simulink model "PROVA_FINALE_LOAD_ARDUINO_15_10_RIF_COSTANTI"  (R2020b)
settings: Solver=FixedStepDiscrete  StartTime=0.0  StopTime=Inf  FixedStep=0.02  RelTol=1e-3  EnableMultiTasking=on
undefined symbols (not defined in the file or in its folder): attuatore_Amax, attuatore_Amin, attuatore_Emax, attuatore_Emin, attuatore_Rmax, attuatore_Rmin, attuatore_Tmax, attuatore_Tmin, DiscIntNeverNeededParam, interventoA_05, interventoA_1, interventoE_05, interventoE_1, interventoT, inv_A, inv_comp_h, inv_E, inv_R, inv_T, K_AW_B_AP_quota, K_AW_B_becc, K_AW_B_imb, K_AW_B_roll, K_imb_inv, Kd_h_app, Kd_h_flare, Ki_AP_quota_select, Ki_AP_rotta, Ki_AP_vel, Ki_becch, Ki_h_app, Ki_h_cruise, Ki_h_flare, Ki_roll, Kp_AP_quota_hold_h, Kp_AP_quota_hold_l, Kp_AP_quota_select, Kp_AP_rotta, Kp_AP_vel, Kp_becch, Kp_comp_h, Kp_h_app_max, Kp_h_app_min, Kp_h_cruise, Kp_h_flare, Kp_imb, Kp_p, Kp_q, Kp_roll, Kp_Rotta_ATO, Newton, phi_max, phi_min, Raphson, safe_phi, safe_V, t_AP, theta_max, theta_min, time_alarm_SAFE ... (+5)
libraries: simulink_extras x34, arduinolib x24, pid_lib x8, simulink x3, dspsigops x3, svdutilitieslib x3, aerolibtransform2sys x2, aerolibtransform2 x2
(part 2 of 7)

== system PROVA_FINALE_LOAD_ARDUINO_15_10_RIF_COSTANTI/AIR TX/IMU & Attidude ==
  note: NB.: se non si posside un dato inserire una costante con valore 0. I dati vanno messi tutti anche se zeri nell'ordine elencato
  note: Vanno inseriti i collegamenti con i dati provenienti dal sensore inerziale (MTi)
      | in uscita bisogna dare un vettore di 12 componenti contente in ordine:
      | - 3 accelerazioni (x,y,z)
      | - 3 giroscopiche (p,q,r)
      | - 3 comp. campo magnetico
      | -3 angoli di eulero
  AHRS1 : Inport
  Bus Selector : BusSelector  OutputSignals=acc,p,q,r,phi,theta,psi
  Constant : Constant  Value=0  OutDataTypeStr=double  SampleTime=t_AP
  Constant1 : Constant  Value=0  OutDataTypeStr=double  SampleTime=t_AP
  Constant2 : Constant  Value=0  OutDataTypeStr=double  SampleTime=t_AP
  Data Type Conversion : DataTypeConversion  OutDataTypeStr=int16  RndMeth=Simplest
  Data Type Conversion1 : DataTypeConversion  OutDataTypeStr=single
  Gain : Gain  Gain=10^3
  Mux{1,3..5} (4 alike) : Mux  Inputs=3
  Mux2 : Mux  Inputs=2
  IMU : Outport  VectorParamsAs1DForOutWhenUnconnected=off
  ATT : Outport  Port=2  VectorParamsAs1DForOutWhenUnconnected=off
  wires:
  Constant/1 -> Mux5/1
  Mux4/1 -> Mux2/1
  Bus Selector/7 -> Mux4/3  "<psi>"
  Bus Selector/6 -> Mux4/2  "<theta>"
  Bus Selector/5 -> Mux4/1  "<phi>"
  Mux3/1 -> Mux2/2, Mux1/2
  Bus Selector/4 -> Mux3/3  "<r>"
  Bus Selector/3 -> Mux3/2  "<q>"
  Bus Selector/2 -> Mux3/1  "<p>"
  Bus Selector/1 -> Mux1/1  "<acc>"
  AHRS1/1 -> Bus Selector/1
  Mux2/1 -> Data Type Conversion1/1
  Gain/1 -> Data Type Conversion/1
  Data Type Conversion1/1 -> ATT/1
  Data Type Conversion/1 -> IMU/1
  Mux1/1 -> Gain/1
  Constant1/1 -> Mux5/2
  Mux5/1 -> Mux1/3
  Constant2/1 -> Mux5/3

== system PROVA_FINALE_LOAD_ARDUINO_15_10_RIF_COSTANTI/AIR TX/If_subsystem ==
  note: Blocco per la temporizzazione dell'invio dei messaggi
  Data Type Conversion3 : DataTypeConversion  OutDataTypeStr=uint32  RndMeth=Simplest
  Gain : Gain  Gain=100
  Subsystem : Subsystem
  iflogic_function : MATLAB Function  TreatAsAtomicUnit=on
  iflogic : Outport  VectorParamsAs1DForOutWhenUnconnected=off
  time : Outport  Port=2  VectorParamsAs1DForOutWhenUnconnected=off
  wires:
  Subsystem/3(time) -> Gain/1
  Subsystem/2(H_10) -> iflogic_function/2(H10)
  Subsystem/1(H_50) -> iflogic_function/1(H50)
  Gain/1 -> Data Type Conversion3/1
  Data Type Conversion3/1 -> time/1
  iflogic_function/1(iflogic) -> iflogic/1

== system PROVA_FINALE_LOAD_ARDUINO_15_10_RIF_COSTANTI/AIR TX/Servo ==
  note: NB.: se non si posside un dato inserire una costante con valore 0. I dati vanno messi tutti anche se zeri nell'ordine elencato
  note: Vanno inseriti i collegamenti con i dati provenienti dal sensore di velocità
      | in uscita bisogna dare 1 segnale composto da:
      |
      | -  PORT
      | -8 servo
  note: La quota lidar la invio come componente 8 dei servi
  Sensor : Inport
  Servo : Inport  Port=2
  Bus Selector : BusSelector  OutputSignals=Manetta,Equilibratore,Alettoni,Timone
  Bus Selector1 : BusSelector  OutputSignals=quota_lidar
  Constant : Constant  Value=4
  Constant1 : Constant  Value=zeros(3,1)
  Conversione : Subsystem
  Data Type Conversion1 : DataTypeConversion  OutDataTypeStr=uint16  RndMeth=Simplest
  Gain : Gain  Gain=100
  Mux : Mux  Inputs=7
  Saturation : Saturate  UpperLimit=4000  LowerLimit=0
  Servo_data : Outport  VectorParamsAs1DForOutWhenUnconnected=off
  wires:
  Conversione/4(Out4) -> Mux/5
  Conversione/3(Out3) -> Mux/4
  Conversione/2(Out2) -> Mux/3
  Conversione/1(Out1) -> Mux/2
  Bus Selector/1 -> Conversione/1(Manetta)  "<Manetta>"
  Bus Selector/4 -> Conversione/4(Timone)  "<Timone>"
  Bus Selector/3 -> Conversione/3(Alettoni)  "<Alettoni>"
  Bus Selector/2 -> Conversione/2(Equilibratore)  "<Equilibratore>"
  Constant1/1 -> Mux/6
  Constant/1 -> Mux/1
  Servo/1 -> Bus Selector/1
  Mux/1 -> Data Type Conversion1/1
  Data Type Conversion1/1 -> Servo_data/1  "Heading"
  Sensor/1 -> Bus Selector1/1
  Bus Selector1/1 -> Gain/1  "<quota_lidar>"
  Gain/1 -> Saturation/1
  Saturation/1 -> Mux/7

== system PROVA_FINALE_LOAD_ARDUINO_15_10_RIF_COSTANTI/AIR TX/SystemStatus ==
  note: coefficiente moltiplicativo Mavlink
  note: conversione
      | Amper - milliAmper
  note: NB.: se non si posside un dato inserire una costante con valore 0 (se non indicato diversamente sopra).
      | I dati vanno messi tutti anche se zeri nell'ordine elencato
  note: Vanno inseriti i collegamenti con i dati provenienti dal autopilota
      | in uscita bisogna dare 4 segnali:
      |
      | -onboard_control_sensor_present
      | - vettore con: load, voltaggio batteria(millivolt), drop rate, 5 flag di errore
      | -corrente della batteria (10*milliamper) -1 se non noto
      | -batteria rimanente (in percentuale) -1 se non noto
  note: conversione
      | Amper - milliAmper
  SyS_input : Inport
  Alarm : Inport  Port=2
  batteria : Inport  Port=3
  " " : Constant  Value=0  OutDataTypeStr=uint16
  Data Type Conversion : DataTypeConversion  OutDataTypeStr=uint32
  Data Type Conversion1 : DataTypeConversion  OutDataTypeStr=int16
  Data Type Conversion2 : DataTypeConversion  OutDataTypeStr=uint16
  Data Type Conversion3 : DataTypeConversion  OutDataTypeStr=int8
  Data Type Conversion4 : DataTypeConversion  OutDataTypeStr=uint16
  Demux : Demux  Outputs=3
  Gain : Gain  Gain=1000  OutDataTypeStr=uint16
  Gain1 : Gain  Gain=0.1  OutDataTypeStr=int16
  Gain2 : Gain  Gain=1000  OutDataTypeStr=int16
  Mux : Mux  Inputs=5
  load uint16 : Constant  Value=10  OutDataTypeStr=uint16
  onboard_control_sensor_present uint32 : Constant  Value=[1; 1 ;1]  OutDataTypeStr=uint32
  onboard : Outport  VectorParamsAs1DForOutWhenUnconnected=off
  LVDE : Outport  Port=2  VectorParamsAs1DForOutWhenUnconnected=off
  B_current : Outport  Port=3  VectorParamsAs1DForOutWhenUnconnected=off
  B_remaining : Outport  Port=4  VectorParamsAs1DForOutWhenUnconnected=off
  wires:
  Gain2/1 -> Gain1/1
  Demux/3 -> Gain2/1
  Gain1/1 -> Data Type Conversion1/1
  Demux/1 -> Gain/1
  batteria/1 -> Demux/1
  " "/1 -> Mux/4
  Data Type Conversion4/1 -> Mux/5
  Alarm/1 -> Data Type Conversion4/1
  SyS_input/1 -> Mux/3
  Data Type Conversion3/1 -> B_remaining/1  "B_Remaining"
  Data Type Conversion1/1 -> B_current/1  "B_Current"
  Data Type Conversion2/1 -> LVDE/1  "LVDE"
  Data Type Conversion/1 -> onboard/1  "onboard"
  Demux/2 -> Data Type Conversion3/1
  Mux/1 -> Data Type Conversion2/1
  Gain/1 -> Mux/2
  load uint16/1 -> Mux/1
  onboard_control_sensor_present uint32/1 -> Data Type Conversion/1

== system PROVA_FINALE_LOAD_ARDUINO_15_10_RIF_COSTANTI/AIR TX/VFR ==
  note: NB.: se non si posside un dato inserire una costante con valore 0. I dati vanno messi tutti anche se zeri nell'ordine elencato
  note: Vanno inseriti i collegamenti con i dati provenienti dal sensore di velocità
      | in uscita bisogna dare 3 segnali:
      |
      | -  AGAC: airspeed, groundspeed,altitudine, rateo salita
      | -Heading
      | -Throttle: spinta o rpm del motore
  note: inserire 100/massimo valore
      | deve uscire una percentuale
      | FISSATO PER QUOTA IL 5-5-2016
  VFR1 : Inport
  Bus Selector : BusSelector  OutputSignals=Tas,Alt,RC,heading,RPM
  Data Type Conversion : DataTypeConversion  OutDataTypeStr=single
  Data Type Conversion1 : DataTypeConversion  OutDataTypeStr=int16  RndMeth=Simplest
  Data Type Conversion2 : DataTypeConversion  OutDataTypeStr=uint16  RndMeth=Simplest
  Mux : Mux
  Radians to Degrees : simulink_extras/Transformations/Radians to Degrees
  USCITA PERCENTUALE : Gain  Gain=100/9000
  airspeed groundspeed alt climb1 : Constant  Value=0  OutDataTypeStr=double  SampleTime=t_AP
  wrapTo360 : Subsystem
  AGAC : Outport  VectorParamsAs1DForOutWhenUnconnected=off
  Heading : Outport  Port=2  VectorParamsAs1DForOutWhenUnconnected=off
  Throttle : Outport  Port=3  VectorParamsAs1DForOutWhenUnconnected=off
  wires:
  Mux/1 -> Data Type Conversion/1
  Bus Selector/5 -> USCITA PERCENTUALE/1  "<RPM>"
  Bus Selector/4 -> Radians to Degrees/1  "<heading>"
  Bus Selector/3 -> Mux/4  "<RC>"
  Bus Selector/2 -> Mux/3  "<Alt>"
  Bus Selector/1 -> Mux/1  "<Tas>"
  airspeed groundspeed alt climb1/1 -> Mux/2
  VFR1/1 -> Bus Selector/1
  Data Type Conversion2/1 -> Throttle/1  "Throttle"
  Data Type Conversion1/1 -> Heading/1  "Heading"
  Data Type Conversion/1 -> AGAC/1  "AGAC"
  USCITA PERCENTUALE/1 -> Data Type Conversion2/1
  Radians to Degrees/1 -> wrapTo360/1(In1)
  wrapTo360/1(Out1) -> Data Type Conversion1/1  "uscita"

== system PROVA_FINALE_LOAD_ARDUINO_15_10_RIF_COSTANTI/AIR TX/Waypoints ==
  GC_req : Inport
  "Sensori " : Inport  Port=2
  Bus Selector : BusSelector  OutputSignals=Alt
  Bus Selector3 : BusSelector  OutputSignals=Val_float,WP_db_info,WP_db_param,GC_info
  MATLAB Function : MATLAB Function  TreatAsAtomicUnit=on
  Terminator : Terminator
  GC_info : Outport  VectorParamsAs1DForOutWhenUnconnected=off
  P_value : Outport  Port=2  VectorParamsAs1DForOutWhenUnconnected=off
  WP_info : Outport  Port=3  VectorParamsAs1DForOutWhenUnconnected=off
  WP_param : Outport  Port=4  VectorParamsAs1DForOutWhenUnconnected=off
  wires:
  "Sensori "/1 -> Bus Selector/1
  Bus Selector3/1 -> P_value/1  "<Val_float>"
  Bus Selector/1 -> Terminator/1  "<Alt>"
  MATLAB Function/2(WP_param) -> WP_param/1
  Bus Selector3/3 -> MATLAB Function/2(WP_param_in)  "<WP_db_param>"
  MATLAB Function/1(WP_info) -> WP_info/1
  Bus Selector3/2 -> MATLAB Function/1(WP_info_in)  "<WP_db_info>"
  Bus Selector3/4 -> MATLAB Function/3(GC_info), GC_info/1  "<GC_info>"
  GC_req/1 -> Bus Selector3/1

== system PROVA_FINALE_LOAD_ARDUINO_15_10_RIF_COSTANTI/AUTOPILOTA/AUTOPILOTI1 ==
  Sensori : Inport
  Parametri Sistema di Controllo : Inport  Port=2
  Riferimenti : Inport  Port=3
  Riferimenti Safe : Inport  Port=4
  Alarm Safe : Inport  Port=5
  comandi : Inport  Port=6
  Switch attuatori : Inport  Port=7
  Switch_ATO : Inport  Port=8
  Switch_AL : Inport  Port=9
  traking theta : Inport  Port=10
  manetta_track : Inport  Port=11
  track_phi : Inport  Port=12
  Bus Creator : BusCreator  Inputs=2
  Bus Selector : BusSelector  OutputSignals=switch_manetta,switch_alettoni
  Bus Selector2 : BusSelector  OutputSignals=throttle_safe,theta_safe,phi_safe
  CONTROLLORE DI QUOTA : Subsystem
  CONTROLLORE DI ROTTA : Subsystem
  CONTROLLORE DI VELOCITA' : Subsystem
  Switch di selezione riferimeti per i loop interni 1 : MultiPortSwitch  DataPortOrder=Zero-based contiguous  Inputs=2  zeroidx=on
  Switch di selezioneriferimeti per i loop interni 2 : MultiPortSwitch  DataPortOrder=Zero-based contiguous  Inputs=2  zeroidx=on
  Switch di selezioneriferimeti per i loop interni 3 : MultiPortSwitch  DataPortOrder=Zero-based contiguous  Inputs=2  zeroidx=on
  Riferimento Manetta : Outport  VectorParamsAs1DForOutWhenUnconnected=off
  Riferimenti Rollio e Beccheggio : Outport  Port=2  VectorParamsAs1DForOutWhenUnconnected=off
  tag scope: alarm_safe=global, phi_safe=global, theta_safe=global, throttle_safe=global
  wires:
  Bus Creator/1 -> Riferimenti Rollio e Beccheggio/1  "Rif_loop_int"
  CONTROLLORE DI VELOCITA'/1(Riferimento Manetta) -> Switch di selezione riferimeti per i loop interni 1/2  "Riferimento Manetta"
  Switch di selezione riferimeti per i loop interni 1/1 -> Riferimento Manetta/1  "Riferimento Manetta"
  Switch di selezioneriferimeti per i loop interni 2/1 -> Bus Creator/1  "theta_rif"
  Switch di selezioneriferimeti per i loop interni 3/1 -> Bus Creator/2  "phi_rif"
  [alarm_safe] -> Switch di selezioneriferimeti per i loop interni 2/1
  [alarm_safe] -> Switch di selezioneriferimeti per i loop interni 3/1
  Sensori/1 -> CONTROLLORE DI VELOCITA'/1(Sensori), CONTROLLORE DI ROTTA/2(Sensori), CONTROLLORE DI QUOTA/1(Sensori)
  Riferimenti/1 -> CONTROLLORE DI ROTTA/1(Riferimenti), CONTROLLORE DI QUOTA/2(Riferimenti), CONTROLLORE DI VELOCITA'/2(Riferimenti)
  Parametri Sistema di Controllo/1 -> CONTROLLORE DI VELOCITA'/3(Parametri Sistema di Controllo), CONTROLLORE DI QUOTA/3(Parametri Sistema di Controllo), CONTROLLORE DI ROTTA/3(Parametri Sistema di Controllo)
  Riferimenti Safe/1 -> Bus Selector2/1
  Alarm Safe/1 -> [alarm_safe]
  Bus Selector2/1 -> [throttle_safe]  "<throttle_safe>"
  Bus Selector2/2 -> [theta_safe]  "<theta_safe>"
  Bus Selector2/3 -> [phi_safe]  "<phi_safe>"
  [alarm_safe] -> Switch di selezione riferimeti per i loop interni 1/1
  [throttle_safe] -> Switch di selezione riferimeti per i loop interni 1/3
  [theta_safe] -> Switch di selezioneriferimeti per i loop interni 2/3
  [phi_safe] -> Switch di selezioneriferimeti per i loop interni 3/3
  Switch attuatori/1 -> Bus Selector/1
  Bus Selector/1 -> [switch_manetta]  "<switch_manetta>"
  Bus Selector/2 -> [switch_alettoni]  "<switch_alettoni>"
  comandi/1 -> CONTROLLORE DI VELOCITA'/5(comandi)
  [switch_manetta] -> CONTROLLORE DI VELOCITA'/4(switch_manetta)
  [switch_alettoni] -> CONTROLLORE DI ROTTA/4("switch alettoni ")
  CONTROLLORE DI ROTTA/1(phi_rif) -> Switch di selezioneriferimeti per i loop interni 3/2  "phi_rif"
  Switch_ATO/1 -> [Switch_ATO]
  Switch_AL/1 -> [Switch_AL]
  [Switch_AL] -> CONTROLLORE DI VELOCITA'/6(Switch_AL)
  CONTROLLORE DI QUOTA/1(theta_rif) -> Switch di selezioneriferimeti per i loop interni 2/2  "theta_rif"
  [Switch_ATO] -> CONTROLLORE DI QUOTA/4(Ato)
  traking theta/1 -> CONTROLLORE DI QUOTA/5(traking_theta)
  manetta_track/1 -> CONTROLLORE DI VELOCITA'/7(manetta_track)
  track_phi/1 -> CONTROLLORE DI ROTTA/5(track_phi)
  [Switch_ATO] -> CONTROLLORE DI ROTTA/6(Switch_ATO)

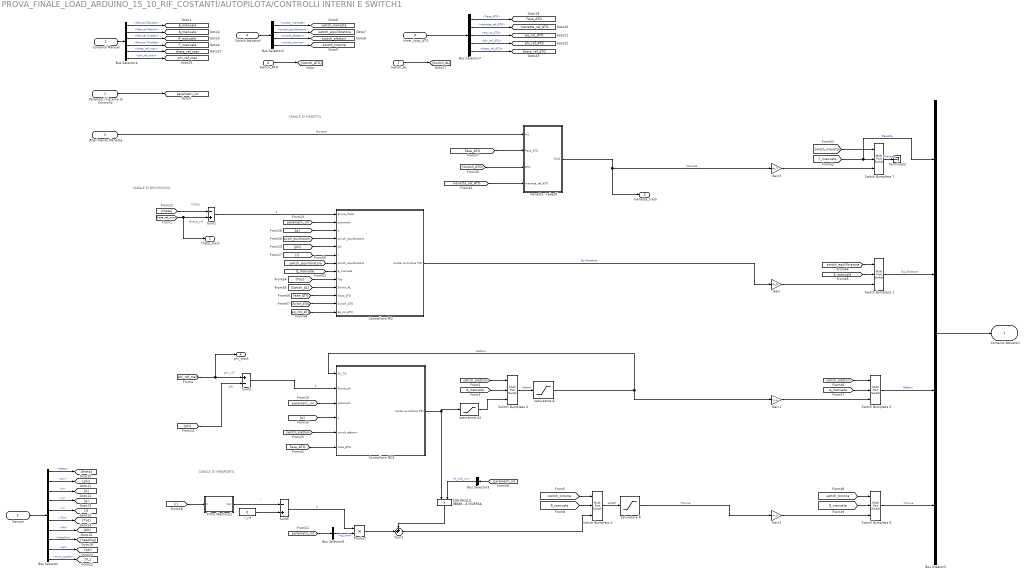
== system PROVA_FINALE_LOAD_ARDUINO_15_10_RIF_COSTANTI/AUTOPILOTA/CONTROLLI INTERNI E SWITCH1 ==
  note: CANALE DI
      |  MANETTA
  note: theta
  note: theta_rif
  note: CANALE DI
      |  BECCHEGGIO
  note: CANALE
      | DI IMBARDATA
  note: phi
  note: phi_rif
  note: r
  Parametri Sistema di Controllo : Inport
  Comandi Manuali : Inport  Port=2
  Riferimento Manetta : Inport  Port=3
  Switch Attuatori : Inport  Port=4
  Sensori : Inport  Port=5
  Switch_ATO : Inport  Port=6
  Switch_AL : Inport  Port=7
  Inner_loop_ATO : Inport  Port=8
  "  CONTROLLO IMBARDATA INVERSA" : Product  RndMeth=Zero
  Bus Creator3 : BusCreator  Inputs=4
  Bus Selector : BusSelector  OutputSignals=theta,phi,p,q,r,Tas,Alt,heading,psi,horiz_speed
  Bus Selector2 : BusSelector  OutputSignals=switch_manetta,switch_equilibratore,switch_alettoni,switch_timone
  Bus Selector3 : BusSelector  OutputSignals=K_imb_inv
  Bus Selector4 : BusSelector  OutputSignals=Manual Elevator,Manual Aileron,Manual Rudder,Manual Throttle,theta_ref_man,phi_ref_man
  Bus Selector5 : BusSelector  OutputSignals=Kp_imb
  Bus Selector7 : BusSelector  OutputSignals=Fase_ATO,manetta_ref_ATO,eq_rot_ATO,phi_ref_ATO,theta_ref_ATO
  Controllore PID : Subsystem
  Controllore PID1 : Subsystem
  Filtro Washout1 : Subsystem
  Gain : Gain  Gain=inv_E
  Gain1 : Gain  Gain=inv_A
  Gain2 : Gain  Gain=inv_R
  Gain3 : Gain  Gain=inv_T
  Product : Product  RndMeth=Zero
  Sum1 : Sum  Inputs=++|
  Sum2 : Sum  Inputs=-+
  Sum5 : Sum  Inputs=+-
  Sum9 : Sum  Inputs=-+
  Switch Bumpless {1,3..7} (6 alike) : MultiPortSwitch  DataPortOrder=Zero-based contiguous  Inputs=2  zeroidx=on
  Terminator : Terminator
  manetta - takeoff : Subsystem
  r_rif : Constant  Value=0
  saturatore A : Saturate  UpperLimit=attuatore_Amax  LowerLimit=attuatore_Amin
  saturatore A1 : Saturate  UpperLimit=attuatore_Amax  LowerLimit=attuatore_Amin
  saturatore R : Saturate  UpperLimit=attuatore_Rmax  LowerLimit=attuatore_Rmin
  Comandi Attuatori : Outport  VectorParamsAs1DForOutWhenUnconnected=off
  theta_track : Outport  Port=2  VectorParamsAs1DForOutWhenUnconnected=off
  manetta_track : Outport  Port=3  VectorParamsAs1DForOutWhenUnconnected=off
  phi_track : Outport  Port=4  VectorParamsAs1DForOutWhenUnconnected=off
  tag scope: A_manuale=global, E_manuale=global, Fase_ATO=global, R_manuale=global, T_manuale=global, eq_rot_ATO=global, manetta_ref_ATO=global, parametri_int=global, phi_ref_ATO=global, phi_ref_man=global, switch_alettoni=global, switch_equilibratore=global, switch_manetta=global, switch_timone=global, theta_ref_ATO=global, theta_ref_man=global
  wires:
  Comandi Manuali/1 -> Bus Selector4/1
  Bus Selector4/1 -> [E_manuale]  "<Manual Elevator>"
  Bus Selector4/2 -> [A_manuale]  "<Manual Aileron>"
  Bus Selector4/3 -> [R_manuale]  "<Manual Rudder>"
  Bus Selector4/4 -> [T_manuale]  "<Manual Throttle>"
  Parametri Sistema di Controllo/1 -> [parametri_int]
  Switch Attuatori/1 -> Bus Selector2/1
  Bus Selector2/1 -> [switch_manetta]  "<switch_manetta>"
  Bus Selector2/2 -> [switch_equilibratore]  "<switch_equilibratore>"
  Bus Selector2/3 -> [switch_alettoni]  "<switch_alettoni>"
  Bus Selector2/4 -> [switch_timone]  "<switch_timone>"
  Sensori/1 -> Bus Selector/1
  Switch Bumpless 3/1 -> saturatore A/1  "deltaA"
  saturatore A/1 -> Gain1/1, Controllore PID1/1(Err_Trk)  "Alettoni"
  [switch_alettoni] -> Switch Bumpless 3/1
  [A_manuale] -> Switch Bumpless 3/2
  [switch_timone] -> Switch Bumpless 4/1
  [R_manuale] -> Switch Bumpless 4/2
  r_rif/1 -> Sum9/2
  Filtro Washout1/1(Out) -> Sum9/1
  Bus Creator3/1 -> Comandi Attuatori/1
  Bus Selector3/1 -> "  CONTROLLO IMBARDATA INVERSA"/2  "<K_imb_inv>"
  [parametri_int] -> Bus Selector3/1
  Sum2/1 -> Controllore PID/1(Errore_theta)  "e"
  [switch_equilibratore] -> Controllore PID/4("switch_equilibratore ")
  saturatore A1/1 -> Switch Bumpless 3/3
  [parametri_int] -> Controllore PID/2(parametri)
  [parametri_int] -> Controllore PID1/3(parametri)
  Sum5/1 -> Controllore PID1/2(Errore_phi)  "e"
  Controllore PID1/1(Uscita controllore PID) -> saturatore A1/1, "  CONTROLLO IMBARDATA INVERSA"/1
  saturatore R/1 -> Gain2/1  "Timone"
  Switch Bumpless 4/1 -> saturatore R/1  "deltaR"
  Sum9/1 -> Product/1  "e"
  [parametri_int] -> Bus Selector5/1
  Bus Selector5/1 -> Product/2  "<Kp_imb>"
  Product/1 -> Sum1/2
  "  CONTROLLO IMBARDATA INVERSA"/1 -> Sum1/1
  Switch_ATO/1 -> [Switch_ATO]
  Bus Selector/6 -> [Tas]  "<Tas>"
  Bus Selector/7 -> [Alt]  "<Alt>"
  Sum1/1 -> Switch Bumpless 4/3
  Switch_AL/1 -> [Switch_AL]
  Controllore PID/1(Uscita controllore PID) -> Gain/1  "Equilibratore"
  [phi_ref_man] -> phi_track/1, Sum5/1
  Inner_loop_ATO/1 -> Bus Selector7/1
  Bus Selector7/1 -> [Fase_ATO]  "<Fase_ATO>"
  Bus Selector7/2 -> [manetta_ref_ATO]  "<manetta_ref_ATO>"
  Bus Selector7/3 -> [eq_rot_ATO]  "<eq_rot_ATO>"
  Bus Selector7/4 -> [phi_ref_ATO]  "<phi_ref_ATO>"
  Bus Selector7/5 -> [theta_ref_ATO]  "<theta_ref_ATO>"
  manetta - takeoff/1(Out1) -> Gain3/1, manetta_track/1  "Manetta"
  Riferimento Manetta/1 -> manetta - takeoff/1(In1)  "Manetta"
  [switch_alettoni] -> Controllore PID1/5("switch_alettoni ")
  [theta] -> Sum2/1
  Bus Selector/1 -> [theta]  "<theta>"
  [phi] -> Controllore PID/5("phi ")
  [phi] -> Sum5/2
  Bus Selector/2 -> [phi]  "<phi>"
  [p] -> Controllore PID1/4("p ")
  Bus Selector/3 -> [p]  "<p>"
  [q] -> Controllore PID/3("q ")
  Bus Selector/4 -> [q]  "<q>"
  [r] -> Controllore PID/6(r)
  [r] -> Filtro Washout1/1(In)
  Bus Selector/5 -> [r]  "<r>"
  Bus Selector/9 -> [psi]  "<psi>"
  [Switch_ATO] -> manetta - takeoff/3(ATO)
  [Fase_ATO] -> manetta - takeoff/2(Fase_ATO)
  [manetta_ref_ATO] -> manetta - takeoff/4(manetta_ref_ATO)
  [Fase_ATO] -> Controllore PID1/6(Fase_ATO)
  Bus Selector/8 -> [heading]  "<heading>"
  Bus Selector/10 -> [V_]  "<horiz_speed>"
  Switch Bumpless 1/1 -> Bus Creator3/2  "Equilibratore"
  [E_manuale] -> Switch Bumpless 1/2
  [switch_equilibratore] -> Switch Bumpless 1/1
  Gain/1 -> Switch Bumpless 1/3
  [switch_alettoni] -> Switch Bumpless 5/1
  [A_manuale] -> Switch Bumpless 5/2
  Switch Bumpless 5/1 -> Bus Creator3/3  "Alettoni"
  Gain1/1 -> Switch Bumpless 5/3
  [switch_timone] -> Switch Bumpless 6/1
  [R_manuale] -> Switch Bumpless 6/2
  Switch Bumpless 6/1 -> Bus Creator3/4  "Timone"
  Gain2/1 -> Switch Bumpless 6/3
  [switch_manetta] -> Switch Bumpless 7/1
  [T_manuale] -> Bus Creator3/1, Switch Bumpless 7/2  "Manetta"
  Gain3/1 -> Switch Bumpless 7/3
  [switch_equilibratore] -> Controllore PID/7(switch_equilibratore)
  [E_manuale] -> Controllore PID/8(E_manuale)
  [Switch_AL] -> Controllore PID/10(Switch_AL)
  [Tas] -> Controllore PID/9(Tas)
  [Fase_ATO] -> Controllore PID/11(Fase_ATO)
  [Switch_ATO] -> Controllore PID/12(Switch_ATO)
  [eq_rot_ATO] -> Controllore PID/13(Eq_rot_ATO)
  Bus Selector4/6 -> [phi_ref_man]  "<phi_ref_man>"
  Bus Selector4/5 -> [theta_ref_man]  "<theta_ref_man>"
  [theta_ref_man] -> theta_track/1, Sum2/2
  Switch Bumpless 7/1 -> Terminator/1  "Manetta"

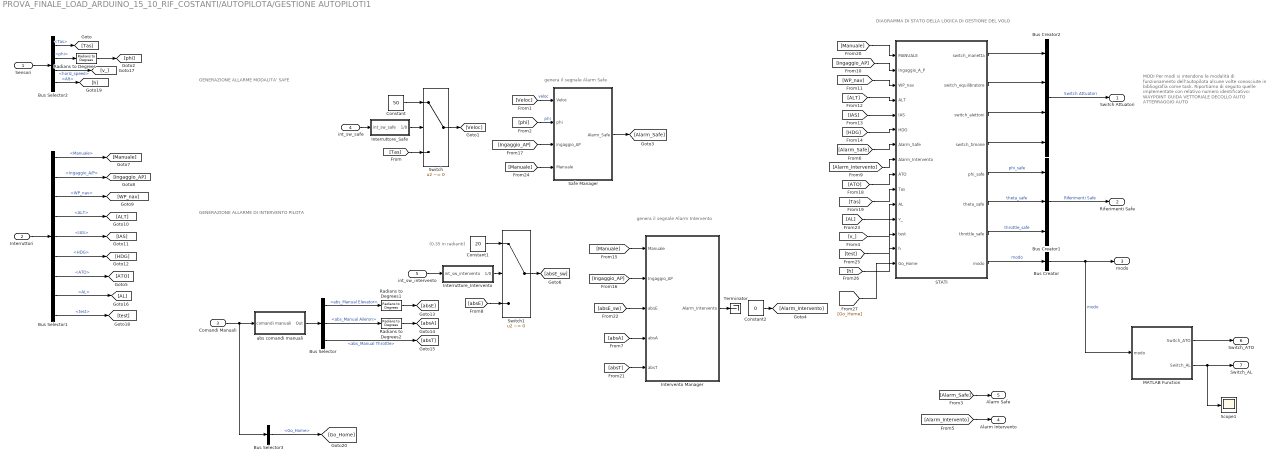
== system PROVA_FINALE_LOAD_ARDUINO_15_10_RIF_COSTANTI/AUTOPILOTA/GESTIONE AUTOPILOTI1 ==
  note: (0.35 in radianti)
  note: GENERAZIONE ALLARME DI INTERVENTO PILOTA
  note: genera il segnale Alarm Safe
  note: genera il segnale Alarm Intervento
  note: GENERAZIONE ALLARME MODALITA' SAFE
  note: DIAGRAMMA DI STATO
      | DELLA LOGICA DI GESTIONE DEL VOLO
  note: MODI
      | Per modi si intendono le modalità di funzionamento dell'autopilota alcune volte conosciute in bibliografia come task. Riportiamo di seguito quelle implementate con relativo numero identificativo:
      |
      | WAYPOINT
      | GUIDA VETTORIALE
      | DECOLLO AUTO
      | ATTERRAGGIO AUTO
  Sensori : Inport
  "Interruttori " : Inport  Port=2
  Comandi Manuali : Inport  Port=3
  int_sw_safe : Inport  Port=4
  int_sw_intervento : Inport  Port=5
  " STATI" : Stateflow chart  TreatAsAtomicUnit=on
  Bus Creator : BusCreator  Inputs=1
  Bus Creator1 : BusCreator  Inputs=3
  Bus Creator2 : BusCreator  Inputs=4
  Bus Selector : BusSelector  OutputSignals=abs_Manual Elevator,abs_Manual Aileron,abs_Manual Throttle
  Bus Selector1 : BusSelector  OutputSignals=Manuale,Ingaggio_A/P,WP_nav,ALT,IAS,HDG,ATO,AL,test
  Bus Selector2 : BusSelector  OutputSignals=Tas,phi,horiz_speed,Alt
  Bus Selector3 : BusSelector  OutputSignals=Go_Home
  Constant : Constant  Value=50
  Constant1 : Constant  Value=20
  Constant2 : Constant  Value=0  SampleTime=0.02
  Interruttore_Intervento : Subsystem
  Interruttore_Safe : Subsystem
  Intervento Manager : Subsystem
  MATLAB Function : MATLAB Function  TreatAsAtomicUnit=on
  Radians to Degrees : simulink_extras/Transformations/Radians to Degrees
  Radians to Degrees1 : simulink_extras/Transformations/Radians to Degrees
  Radians to Degrees2 : simulink_extras/Transformations/Radians to Degrees
  Safe Manager : Subsystem
  Scope1 : Scope
  Switch : Switch  Criteria=u2 ~= 0
  Switch1 : Switch  Criteria=u2 ~= 0
  Terminator : Terminator
  abs comandi manuali : Subsystem
  Switch Attuatori : Outport  VectorParamsAs1DForOutWhenUnconnected=off
  Riferimenti Safe : Outport  Port=2  VectorParamsAs1DForOutWhenUnconnected=off
  modo : Outport  Port=3  VectorParamsAs1DForOutWhenUnconnected=off
  Alarm Intervento : Outport  Port=4  VectorParamsAs1DForOutWhenUnconnected=off
  Alarm Safe : Outport  Port=5  VectorParamsAs1DForOutWhenUnconnected=off
  Switch_ATO : Outport  Port=6  VectorParamsAs1DForOutWhenUnconnected=off
  Switch_AL : Outport  Port=7  VectorParamsAs1DForOutWhenUnconnected=off
  wires:
  "Interruttori "/1 -> Bus Selector1/1
  Bus Selector1/1 -> [Manuale]  "<Manuale>"
  abs comandi manuali/1(Out) -> Bus Selector/1
  Bus Selector/1 -> Radians to Degrees1/1  "<abs_Manual Elevator>"
  Bus Selector/3 -> [absT]  "<abs_Manual Throttle>"
  Comandi Manuali/1 -> Bus Selector3/1, abs comandi manuali/1(comandi manuali)
  Sensori/1 -> Bus Selector2/1
  Bus Selector1/4 -> [ALT]  "<ALT>"
  Bus Selector1/5 -> [IAS]  "<IAS>"
  Bus Selector1/6 -> [HDG]  "<HDG>"
  Bus Selector2/2 -> Radians to Degrees/1  "<phi>"
  Radians to Degrees/1 -> [phi]
  Safe Manager/1(Alarm_Safe) -> [Alarm_Safe]
  Bus Selector/2 -> Radians to Degrees2/1  "<abs_Manual Aileron>"
  Bus Selector1/3 -> [WP_nav]  "<WP_nav>"
  Bus Selector2/1 -> [Tas]  "<Tas>"
  Switch/1 -> [Veloc]
  Constant/1 -> Switch/1
  [Tas] -> Switch/3
  [Veloc] -> Safe Manager/1(Veloc)  "veloc"
  Bus Selector1/2 -> [Ingaggio_AP]  "<Ingaggio_A/P>"
  [phi] -> Safe Manager/2(phi)  "phi"
  Interruttore_Safe/1(1/0) -> Switch/2
  [Alarm_Safe] -> Alarm Safe/1
  Intervento Manager/1(Alarm_Intervento) -> Terminator/1
  [Alarm_Intervento] -> Alarm Intervento/1
  Constant1/1 -> Switch1/1
  [absE] -> Switch1/3
  int_sw_intervento/1 -> Interruttore_Intervento/1(int_sw_intervento)
  Interruttore_Intervento/1(1/0) -> Switch1/2
  [Manuale] -> Intervento Manager/1(Manuale)
  [Ingaggio_AP] -> Intervento Manager/2(Ingaggio_AP)
  [Ingaggio_AP] -> Safe Manager/3(ingaggio_AP)
  [absA] -> Intervento Manager/4(absA)
  int_sw_safe/1 -> Interruttore_Safe/1(int_sw_safe)
  Switch1/1 -> [absE_sw]
  [absE_sw] -> Intervento Manager/3(absE)
  Radians to Degrees1/1 -> [absE]
  Radians to Degrees2/1 -> [absA]
  [absT] -> Intervento Manager/5(absT)
  Bus Selector1/7 -> [ATO]  "<ATO>"
  " STATI"/5(phi_safe) -> Bus Creator1/1  "phi_safe"
  " STATI"/6(theta_safe) -> Bus Creator1/2  "theta_safe"
  " STATI"/7(throttle_safe) -> Bus Creator1/3  "throttle_safe"
  Bus Creator1/1 -> Riferimenti Safe/1  "Riferimenti Safe"
  " STATI"/1(switch_manetta) -> Bus Creator2/1
  " STATI"/2(switch_equilibratore) -> Bus Creator2/2
  " STATI"/3(switch_alettoni) -> Bus Creator2/3
  " STATI"/4(switch_timone) -> Bus Creator2/4
  Bus Creator2/1 -> Switch Attuatori/1  "Switch Attuatori"
  " STATI"/8(modo) -> Bus Creator/1  "modo"
  Bus Creator/1 -> MATLAB Function/1(modo), modo/1  "modo"
  [Alarm_Safe] -> " STATI"/7(Alarm_Safe)
  [Alarm_Intervento] -> " STATI"/8(Alarm_Intervento)
  [Manuale] -> " STATI"/1(MANUALE)
  [Ingaggio_AP] -> " STATI"/2(Ingaggio_A_P)
  [WP_nav] -> " STATI"/3(WP_nav)
  [ALT] -> " STATI"/4(ALT)
  [IAS] -> " STATI"/5(IAS)
  [HDG] -> " STATI"/6(HDG)
  [ATO] -> " STATI"/9(ATO)
  [Tas] -> " STATI"/10(Tas)
  Bus Selector1/8 -> [AL]  "<AL>"
  [AL] -> " STATI"/11(AL)
  Bus Selector2/3 -> [v_]  "<horiz_speed>"
  [v_] -> " STATI"/12(v_)
  [Manuale] -> Safe Manager/4(Manuale)
  Bus Selector1/9 -> [test]  "<test>"
  [test] -> " STATI"/13(test)
  MATLAB Function/1(Switch_ATO) -> Switch_ATO/1
  MATLAB Function/2(Switch_AL) -> Scope1/1, Switch_AL/1
  Bus Selector2/4 -> [h]  "<Alt>"
  [h] -> " STATI"/14(h)
  Bus Selector3/1 -> [Go_Home]  "<Go_Home>"
  [Go_Home] -> " STATI"/15(Go_Home)
  Constant2/1 -> [Alarm_Intervento]

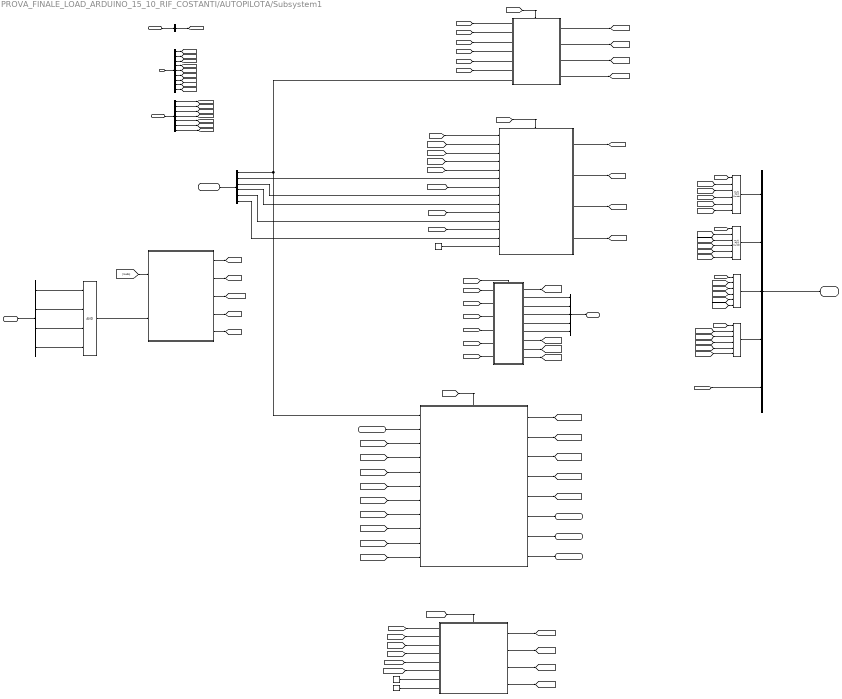
== system PROVA_FINALE_LOAD_ARDUINO_15_10_RIF_COSTANTI/AUTOPILOTA/Subsystem1 ==
  note: MODO 1 : WAYPOINTS
  note: MODO 2 : VETTORIALE
  note: MODO 3 : DECOLLO AUTO
  note: MODO 4 : ATTERRAGGIO AUTO
  note: MODO 5 : GO HOME
  sensori : Inport
  Interruttori : Inport  Port=2
  waypoints e riferimenti vettoriali : Inport  Port=3
  modo : Inport  Port=4
  Cal_home : Inport  Port=5
  Switch_attuatori : Inport  Port=6
  AND : Logic  Inputs=4  IconShape=distinctive  AllPortsSameDT=off  OutDataTypeStr=boolean
  Bus Creator : BusCreator  Inputs=5
  Bus Creator2 : BusCreator  Inputs=5
  Bus Selector : BusSelector  OutputSignals=Lat,Long,Alt,psi,heading,Tas,horiz_speed,psi,theta
  Bus Selector1 : BusSelector  OutputSignals=GC_info,IAS,ALT,HDG,RC,Ingaggio_A/P
  Bus Selector2 : BusSelector  OutputSignals=WP_db_param,WP_db_info,ROTTA,VELOCITA,QUOTA,RC,WP_AL
  Bus Selector3 : BusSelector  OutputSignals=modo
  Bus Selector4 : BusSelector  OutputSignals=switch_manetta,switch_equilibratore,switch_alettoni,switch_timone
  Chart : Stateflow chart  TreatAsAtomicUnit=on
  Constant : Constant  Value=70
  Constant1 : Constant  Value=20
  DECOLLO AUTOMATICO : Subsystem
  RC_default : Constant  Value=2
  Subsystem : Subsystem
  Subsystem1 : Subsystem
  Subsystem2 : Subsystem
  Subsystem3 : Subsystem
  Switch di selezione Task - Waypoint navigation{,1..3} (4 alike) : MultiPortSwitch  Inputs=5
  H_LAT : Outport  VectorParamsAs1DForOutWhenUnconnected=off
  H_LONG : Outport  Port=2  VectorParamsAs1DForOutWhenUnconnected=off
  H_ALT : Outport  Port=3  VectorParamsAs1DForOutWhenUnconnected=off
  Riferimenti : Outport  Port=4  VectorParamsAs1DForOutWhenUnconnected=off
  Inner_loop_ATO : Outport  Port=5  VectorParamsAs1DForOutWhenUnconnected=off
  wires:
  waypoints e riferimenti vettoriali/1 -> Bus Selector2/1
  Bus Selector2/3 -> [ROTTA]  "<ROTTA>"
  Bus Selector2/4 -> [VELOCITA]  "<VELOCITA>"
  Bus Selector2/5 -> [QUOTA]  "<QUOTA>"
  Bus Selector2/6 -> [RC]  "<RC>"
  modo/1 -> Bus Selector3/1
  Bus Selector2/1 -> [WP_db_param]  "<WP_db_param>"
  Bus Selector2/2 -> [WP_db_info]  "<WP_db_info>"
  sensori/1 -> Bus Selector/1
  Bus Selector/1 -> [Lat]  "<Lat>"
  Bus Selector/2 -> [Long]  "<Long>"
  Bus Selector/3 -> [h]  "<Alt>"
  Bus Selector/4 -> [psi]  "<psi>"
  Bus Selector3/1 -> [modo]  "<modo>"
  Bus Selector/6 -> [Tas]  "<Tas>"
  [Tas] -> DECOLLO AUTOMATICO/1(Tas)
  DECOLLO AUTOMATICO/1(rotta_ATO) -> [rotta_ATO]
  DECOLLO AUTOMATICO/7(h_ref_ATO) -> [h_ATO]
  DECOLLO AUTOMATICO/9(RC_ref_ATO) -> [RC_ATO]
  DECOLLO AUTOMATICO/8(Tas_ref_ATO) -> [V_ATO]
  Interruttori/1 -> Bus Selector1/1
  Bus Selector2/7 -> [WP_AL]  "<WP_AL>"
  Bus Selector/7 -> [V_]  "<horiz_speed>"
  Switch di selezione Task - Waypoint navigation3/1 -> Bus Creator2/4  "ROTTA"
  Bus Creator2/1 -> Riferimenti/1
  Switch di selezione Task - Waypoint navigation/1 -> Bus Creator2/1  "RC"
  Switch di selezione Task - Waypoint navigation1/1 -> Bus Creator2/2  "VELOCITA"
  [modo] -> Switch di selezione Task - Waypoint navigation/1
  [modo] -> Switch di selezione Task - Waypoint navigation1/1
  [modo] -> Switch di selezione Task - Waypoint navigation2/1
  [modo] -> Switch di selezione Task - Waypoint navigation3/1
  [RC_vett] -> Switch di selezione Task - Waypoint navigation/3
  [V_vett] -> Switch di selezione Task - Waypoint navigation1/3
  [rotta_vett] -> Switch di selezione Task - Waypoint navigation3/3
  [RC_wp] -> Switch di selezione Task - Waypoint navigation/2
  [VELOCITA_wp] -> Switch di selezione Task - Waypoint navigation1/2
  [ROTTA_wp] -> Switch di selezione Task - Waypoint navigation3/2
  [V_ATO] -> Switch di selezione Task - Waypoint navigation1/4
  [RC_ATO] -> Switch di selezione Task - Waypoint navigation/4
  [rotta_ATO] -> Switch di selezione Task - Waypoint navigation3/4
  [RC_AL] -> Switch di selezione Task - Waypoint navigation/5
  [V_AL] -> Switch di selezione Task - Waypoint navigation1/5
  [rotta_AL] -> Switch di selezione Task - Waypoint navigation3/5
  [V_goHome] -> Switch di selezione Task - Waypoint navigation1/6
  [rotta_goHome] -> Switch di selezione Task - Waypoint navigation3/6
  [RC_goHome] -> Switch di selezione Task - Waypoint navigation/6
  Bus Selector/5 -> [heading]  "<heading>"
  [landing_selector] -> Bus Creator2/5  "landing_selector"
  Switch di selezione Task - Waypoint navigation2/1 -> Bus Creator2/3  "QUOTA"
  [QUOTA_wp] -> Switch di selezione Task - Waypoint navigation2/2
  [h_vett] -> Switch di selezione Task - Waypoint navigation2/3
  [h_ATO] -> Switch di selezione Task - Waypoint navigation2/4
  [h_AL] -> Switch di selezione Task - Waypoint navigation2/5
  [h_goHome] -> Switch di selezione Task - Waypoint navigation2/6
  [h] -> DECOLLO AUTOMATICO/2(h)
  [modo] -> DECOLLO AUTOMATICO/3(modo)
  Bus Selector/8 -> [psi_imu]  "<psi>"
  [psi_imu] -> DECOLLO AUTOMATICO/4(psi_imu)
  DECOLLO AUTOMATICO/2(Fase_ATO) -> Bus Creator/1  "Fase_ATO"
  DECOLLO AUTOMATICO/3(manetta_ref_ATO) -> Bus Creator/2  "manetta_ref_ATO"
  DECOLLO AUTOMATICO/4(eq_rot_ATO) -> Bus Creator/3  "eq_rot_ATO"
  DECOLLO AUTOMATICO/5(phi_ref_ATO) -> Bus Creator/4  "phi_ref_ATO"
  DECOLLO AUTOMATICO/6(theta_ref_ATO) -> Bus Creator/5  "theta_ref_ATO"
  Bus Creator/1 -> Inner_loop_ATO/1
  Subsystem1/2(QUOTA_AL) -> [h_AL]
  Cal_home/1 -> Subsystem1/2(Cal_home)
  Subsystem1/6(H_LAT) -> H_LAT/1
  Subsystem1/1(TAS_AL) -> [V_AL]
  Subsystem1/7(H_LONG) -> H_LONG/1
  Subsystem1/8(H_ALT) -> H_ALT/1
  Subsystem1/3(RC_AL) -> [RC_AL]
  Subsystem1/5(landing_selector) -> [landing_selector]
  [Lat] -> Subsystem1/3(Lat)
  [Long] -> Subsystem1/4(Long)
  [h] -> Subsystem1/5(h)
  [psi] -> Subsystem1/6(psi)
  [Tas] -> Subsystem1/10(TAS)
  [V_] -> Subsystem1/11(V_)
  [modo] -> Subsystem1/9(modo)
  [WP_db_info] -> Subsystem1/8(wp_db_info)
  [WP_AL] -> Subsystem1/7(wp_al)
  Subsystem1/4(ROTTA_AL) -> [rotta_AL]
  Bus Selector/9 -> [theta]  "<theta>"
  [theta] -> DECOLLO AUTOMATICO/5(theta)
  Bus Selector1/5 -> Subsystem/11(<RC>)  "<RC>"
  [ROTTA] -> Subsystem/2(In2)
  Bus Selector1/2 -> Subsystem/6(<IAS>)  "<IAS>"
  [modo] -> Subsystem/1(In1)
  [QUOTA] -> Subsystem/4(In4)
  Subsystem/2(Out2) -> [h_vett]
  [Vec_selector] -> Subsystem/Enable
  Subsystem/3(Out3) -> [rotta_vett]
  Subsystem/4(Out4) -> [RC_vett]
  Subsystem/1(Out1) -> [V_vett]
  RC_default/1 -> Subsystem/14(In14)
  Bus Selector1/4 -> Subsystem/9(<HDG>)  "<HDG>"
  Bus Selector1/3 -> Subsystem/8(<ALT>)  "<ALT>"
  [RC] -> Subsystem/5(In5)
  [h] -> Subsystem/12(In12)
  [heading] -> Subsystem/7(In7)
  [Tas] -> Subsystem/10(In10)
  Bus Selector1/6 -> Subsystem/13(<Ingaggio_AP>)  "<Ingaggio_A/P>"
  [VELOCITA] -> Subsystem/3(In3)
  Subsystem2/1(RC) -> [RC_wp]
  [WP_db_param] -> Subsystem2/6(In6)
  [WP_db_info] -> Subsystem2/5(In5)
  Subsystem2/2(VELOCITA) -> [VELOCITA_wp]
  Bus Selector1/1 -> Subsystem1/1(<GC_info>), Subsystem2/7(<GC_info>)  "<GC_info>"
  Subsystem2/4(Out4) -> [ROTTA_wp]
  [h] -> Subsystem2/3(In3)
  [Lat] -> Subsystem2/1(In1)
  Subsystem2/3(Out3) -> [QUOTA_wp]
  [Long] -> Subsystem2/2(In2)
  [psi] -> Subsystem2/4(In4)
  [Wp_selector] -> Subsystem2/Enable
  [Ato_selector] -> DECOLLO AUTOMATICO/Enable
  [Al_selector] -> Subsystem1/Enable
  [Lat_Home] -> Subsystem3/5(In5)
  [Long] -> Subsystem3/2(In2)
  [psi] -> Subsystem3/4(In4)
  Constant1/1 -> Subsystem3/8(In8)
  Subsystem3/4(Out4) -> [rotta_goHome]
  [Go_home_selector] -> Subsystem3/Enable
  Constant/1 -> Subsystem3/7(In7)
  Subsystem3/3(Out3) -> [RC_goHome]
  [Long_Home] -> Subsystem3/6(In6)
  Subsystem3/2(Out2) -> [h_goHome]
  [h] -> Subsystem3/3(In3)
  Subsystem3/1(Out1) -> [V_goHome]
  [Lat] -> Subsystem3/1(In1)
  Bus Selector4/1 -> AND/1  "<switch_manetta>"
  Switch_attuatori/1 -> Bus Selector4/1
  Chart/1(Al_selector) -> [Al_selector]
  AND/1 -> Chart/2(Ap_sel)  "Ap_sel"
  Chart/5(Wp_selector) -> [Wp_selector]
  [modo] -> Chart/1(modo)
  Bus Selector4/4 -> AND/4  "<switch_timone>"
  Chart/2(Ato_selector) -> [Ato_selector]
  Bus Selector4/2 -> AND/2  "<switch_equilibratore>"
  Chart/3(Go_home_selector) -> [Go_home_selector]
  Chart/4(Vec_selector) -> [Vec_selector]
  Bus Selector4/3 -> AND/3  "<switch_alettoni>"
  [V_] -> DECOLLO AUTOMATICO/6(V_)

== system PROVA_FINALE_LOAD_ARDUINO_15_10_RIF_COSTANTI/Misure Sensori/ATTOPILOT ==
  note: Il gain 0 - 4095 a 0 - 13.6 V
  note: Il gain 0 - 4095 a 0 - 44.7 A
  Analog Input : arduinolib/Analog Input  pinNumber=6  ReadResultsOnly=off  ConversionTriggerSource=Software  ExternalTriggerType=uint32(0)  OutputDataType=uint16  EnableConversionCompleteNotify=off  EnableOuputStatus=off  SampleTime=t_AP  blockPlatform=arduino
  Analog Input1 : arduinolib/Analog Input  pinNumber=5  ReadResultsOnly=off  ConversionTriggerSource=Software  ExternalTriggerType=uint32(0)  OutputDataType=uint16  EnableConversionCompleteNotify=off  EnableOuputStatus=off  SampleTime=t_AP  blockPlatform=arduino
  Data Type Conversion : DataTypeConversion  OutDataTypeStr=double
  Data Type Conversion1 : DataTypeConversion  OutDataTypeStr=double
  Mux : Mux  Inputs=3
  Scalatura_bit_to_percent_Volt : Subsystem
  m_attopilota_bit_to_current : Gain  Gain=44.7/4095  ParamDataTypeStr=double
  m_attopilota_bit_to_current1 : Gain  Commented=on  Gain=10.9158  ParamDataTypeStr=double
  m_attopilota_bit_to_volt : Gain  Gain=13.6/4095  ParamDataTypeStr=double
  m_attopilota_bit_to_volt1 : Gain  Commented=on  Gain=68/20475  ParamDataTypeStr=double
  misure_Batteria : Outport  VectorParamsAs1DForOutWhenUnconnected=off
  wires:
  Scalatura_bit_to_percent_Volt/1(Percent_Volt) -> Mux/2
  Analog Input/1 -> Data Type Conversion/1
  m_attopilota_bit_to_volt/1 -> Mux/1
  Mux/1 -> misure_Batteria/1
  Data Type Conversion/1 -> m_attopilota_bit_to_volt/1, Scalatura_bit_to_percent_Volt/1(Bit)
  Analog Input1/1 -> Data Type Conversion1/1
  Data Type Conversion1/1 -> m_attopilota_bit_to_current/1
  m_attopilota_bit_to_current/1 -> Mux/3

== system PROVA_FINALE_LOAD_ARDUINO_15_10_RIF_COSTANTI/Misure Sensori/BMP_280 ==
  note: INIZIALIZZAZIONE REGISTRI
      | ATTIVO SOLO ALL'AVVIO DI ARDUINO
  note: Il rate limiter serve ad evitare sbalzi repentini della quota quando si invia la pressione da terra
      | che potrebbero far impazzire il kalman
  note: ACQUISIZIONE MISURE
  note: CALIBRAZIONE ALTIMETRO
  note: FORMULA IPSOMETRICA
  Cal_Alt : Inport
  T_0 : Inport  Port=2
  P_int : Inport  Port=3
  P_ref : Inport  Port=4
  Constant3 : Constant  OutDataTypeStr=boolean  SampleTime=t_AP
  Data Type Conversion : DataTypeConversion  OutDataTypeStr=double
  Data Type Conversion1 : DataTypeConversion
  Data Type Conversion2 : DataTypeConversion  OutDataTypeStr=double
  Dynamic rate limiter : Subsystem
  Execution_loop : Subsystem  TreatAsAtomicUnit=on
  Logical Operator1 : Logic  Operator=NOT  AllPortsSameDT=off  OutDataTypeStr=boolean
  MATLAB Function : MATLAB Function  TreatAsAtomicUnit=on
  MATLAB Function1 : MATLAB Function  TreatAsAtomicUnit=on
  One_time_initialization : Subsystem  TreatAsAtomicUnit=on
  Subsystem : Subsystem
  Unit Delay : UnitDelay  SampleTime=-1  HasFrameUpgradeWarning=on
  h_ : Outport  VectorParamsAs1DForOutWhenUnconnected=off
  P_refer : Outport  Port=2  VectorParamsAs1DForOutWhenUnconnected=off
  P_RAW : Outport  Port=3  VectorParamsAs1DForOutWhenUnconnected=off
  AB_T : Outport  Port=4  VectorParamsAs1DForOutWhenUnconnected=off
  T_0_out : Outport  Port=5  VectorParamsAs1DForOutWhenUnconnected=off
  "pwm_max_min " : Outport  Port=6  VectorParamsAs1DForOutWhenUnconnected=off
  wires:
  One_time_initialization/11(dig_p8) -> Execution_loop/11(Inport7)
  One_time_initialization/4(dig_p1) -> Execution_loop/4(Inport)
  One_time_initialization/7(dig_p4) -> Execution_loop/7(Inport3)
  Execution_loop/2(p) -> Data Type Conversion/1
  Unit Delay/1 -> Execution_loop/Enable, Logical Operator1/1
  One_time_initialization/12(dig_p9) -> Execution_loop/12(Inport8)
  Dynamic rate limiter/1(Y) -> P_refer/1, MATLAB Function1/2(P_ref)
  One_time_initialization/9(dig_p6) -> Execution_loop/9(Inport5)
  One_time_initialization/2(dig_T2) -> Execution_loop/2(Input1)
  One_time_initialization/6(dig_p3) -> Execution_loop/6(Inport2)
  One_time_initialization/10(dig_p7) -> Execution_loop/10(Inport6)
  Logical Operator1/1 -> One_time_initialization/Enable
  One_time_initialization/5(dig_p2) -> Execution_loop/5(Inport1)
  One_time_initialization/3(dig_T3) -> Execution_loop/3(Input2)
  One_time_initialization/1(dig_T1) -> Execution_loop/1(Input)
  Constant3/1 -> Unit Delay/1
  Data Type Conversion/1 -> [P], P_RAW/1, MATLAB Function/2(P)
  One_time_initialization/8(dig_p5) -> Execution_loop/8(Inport4)
  MATLAB Function1/1(h_) -> Data Type Conversion1/1
  Data Type Conversion1/1 -> h_/1
  Execution_loop/1(T) -> AB_T/1, Subsystem/1(T)
  Cal_Alt/1 -> Subsystem/2(Cal_alt)
  Subsystem/2(Cal_alt2) -> MATLAB Function/1(Cal_alt)
  Subsystem/1(T_02) -> MATLAB Function1/1(T_0), T_0_out/1
  T_0/1 -> Subsystem/3(T_01)
  One_time_initialization/13(pwm_max_min) -> "pwm_max_min "/1
  MATLAB Function/2(P_refer) -> Dynamic rate limiter/2(u)
  P_int/1 -> MATLAB Function/3(P_int)
  P_ref/1 -> Data Type Conversion2/1
  MATLAB Function/3(rate_l_dw) -> Dynamic rate limiter/3(lo)
  MATLAB Function/1(rate_l_up) -> Dynamic rate limiter/1(up)
  [P] -> MATLAB Function1/3(P)
  Data Type Conversion2/1 -> MATLAB Function/4(P_cal)

== system PROVA_FINALE_LOAD_ARDUINO_15_10_RIF_COSTANTI/Misure Sensori/GPS_Venus ==
  note: ACQUISIZIONE E DECODIFICA MESSAGGIO
  Cal_alt : Inport
  Demux : Demux  Outputs=6
  Demux1 : Demux  Outputs=2
  Mux : Mux  Inputs=6
  Selector : Selector  InputPortWidth=9  IndexOptions=Index vector (dialog)  Indices=[1 2 3 8 5 6]  OutputSizes=1
  Selector1 : Selector  InputPortWidth=9  IndexOptions=Index vector (dialog)  Indices=[4 7]  OutputSizes=1
  Serial Receive1 : arduinolib/Serial Receive  isARMArch=on  portNumber=0  DataType=uint8  Datalength=32  SampleTime=0.02  showOutStatus=on  blockPlatform=arduino
      settings: SourceProductBaseCode=ARDUINO
  Subsystem1 : Subsystem
  Subsystem2 : Subsystem
  Sum : Sum  Inputs=|+-
  Terminator : Terminator
  Terminator1 : Terminator
  Misure_GPS : Outport  VectorParamsAs1DForOutWhenUnconnected=off
  mario : Outport  Port=2  VectorParamsAs1DForOutWhenUnconnected=off
  wires:
  Serial Receive1/1 -> Subsystem2/1(In1)
  Serial Receive1/2 -> Subsystem2/Enable
  Subsystem2/1(Misure_GPS) -> Selector1/1, Selector/1
  Cal_alt/1 -> Subsystem1/Enable
  Demux/5 -> Mux/5  "heading"
  Demux/3 -> Mux/3  "V"
  Mux/1 -> Misure_GPS/1
  Demux/4 -> Sum/1, Subsystem1/1(h)
  Demux/6 -> Mux/6, Subsystem1/2(fix)
  Demux/2 -> Mux/2  "Long"
  Demux/1 -> Mux/1  "Lat"
  Subsystem1/1(h_to_subtract) -> Sum/2
  Sum/1 -> Mux/4  "quota"
  Selector/1 -> Demux/1
  Selector1/1 -> Demux1/1
  Demux1/1 -> Terminator/1  "Magnetic_declination"
  Demux1/2 -> Terminator1/1  "n_sat"
  Subsystem2/2(mario) -> mario/1

== system PROVA_FINALE_LOAD_ARDUINO_15_10_RIF_COSTANTI/Misure Sensori/MTi ==
  note: MISURE AHRS
  Byte Reversal : svdutilitieslib/Byte Reversal  numInp=1  blockPlatform=arduinoert
      settings: SourceProductBaseCode=ANDROID,ARDUINO,ML_ARDUINO,ECCORTEXA,ECCORTEXR,SC_BEAGLEBONE_BLUE,EC_FREEDOM_BOARD,EC_FRDM_K64F,INTEL_BLOCKSET,JETSONCPU,MICROBIT,NUCLEO,NVIDIA,PX4AUTOPILOTS,RASPPIIO,STMICRODIS,TIC2000,XILINX_BLOCKSET
  Byte Unpack : svdutilitieslib/Byte Unpack  dimensions={[4],[9],[1]}  datatypes={'uint8','single','uint8'}  byteAlign=1  blockPlatform=arduinoert
      settings: SourceProductBaseCode=ANDROID,ARDUINO,ML_ARDUINO,ECCORTEXA,ECCORTEXR,SC_BEAGLEBONE_BLUE,EC_FREEDOM_BOARD,EC_FRDM_K64F,INTEL_BLOCKSET,JETSONCPU,MICROBIT,NUCLEO,NVIDIA,PX4AUTOPILOTS,RASPPIIO,STMICRODIS,TIC2000,XILINX_BLOCKSET
  S-Function Builder : S-Function  InitFcn=try, set_param(gcb,'FunctionName','Mti'), end  FunctionName=Mti  SFunctionModules=Mti_wrapper  SFunctionDeploymentMode=off  EnableBusSupport=off  mask(S-Function Builder){}
      mask help: Simulink:masks:SFunctionBuilder_MD
      mask init: same as PROVA_FINALE_LOAD_ARDUINO_15_10_RIF_COSTANTI/AIR RX/S-Function Builder
      settings: CopyFcn=set_param(gcbh,'LinkStatus','none')  PreSaveFcn=try, set_param(gcb,'FunctionName','Mti'), end  OpenFcn=sfunctionwizard(gcbh)
      mask Display: plot(val(:,1),val(:,2)),disp(sys),port_label('output',1,'messaggio')
  Terminator10 : Terminator
  Terminator9 : Terminator
  Misure MTi : Outport
  wires:
  Byte Unpack/3 -> Terminator10/1
  S-Function Builder/1 -> Byte Unpack/1
  Byte Unpack/1 -> Terminator9/1
  Byte Unpack/2 -> Byte Reversal/1
  Byte Reversal/1 -> Misure MTi/1

== system PROVA_FINALE_LOAD_ARDUINO_15_10_RIF_COSTANTI/RADIOCOMANDO/AILERON ==
  pwm_aileron_max : Inport
  In1 : Inport  Port=2
  pwm_aileron_min : Inport  Port=3
  Constant8 : Constant  Value=attuatore_Amax  OutDataTypeStr=double  SampleTime=-1
  Constant9 : Constant  Value=attuatore_Amin  OutDataTypeStr=double  SampleTime=-1
  Divide : Product  Inputs=*/
  Multiply : Product
  Sum : Sum  Inputs=|+-
  Sum1 : Sum  Inputs=|+-
  Sum2 : Sum  Inputs=|+-
  Sum3 : Sum  Inputs=|++
  Out1 : Outport  VectorParamsAs1DForOutWhenUnconnected=off
  wires:
  Divide/1 -> Multiply/1
  Sum/1 -> Divide/1
  In1/1 -> Sum/1
  Constant8/1 -> Sum2/1
  pwm_aileron_min/1 -> Sum1/2, Sum/2
  pwm_aileron_max/1 -> Sum1/1
  Multiply/1 -> Sum3/1
  Sum2/1 -> Multiply/2
  Constant9/1 -> Sum3/2, Sum2/2
  Sum1/1 -> Divide/2
  Sum3/1 -> Out1/1

== system PROVA_FINALE_LOAD_ARDUINO_15_10_RIF_COSTANTI/RADIOCOMANDO/AILERON1 ==
  pwm_aileron_max : Inport
  In1 : Inport  Port=2
  pwm_aileron_min : Inport  Port=3
  Constant8 : Constant  Value=phi_max  OutDataTypeStr=double  SampleTime=-1
  Constant9 : Constant  Value=phi_min  OutDataTypeStr=double  SampleTime=-1
  Divide : Product  Inputs=*/
  Gain : Gain  Gain=-1
  Multiply : Product
  Saturation : Saturate  UpperLimit=phi_max  LowerLimit=phi_min
  Sum : Sum  Inputs=|+-
  Sum1 : Sum  Inputs=|+-
  Sum2 : Sum  Inputs=|+-
  Sum3 : Sum  Inputs=|++
  Out1 : Outport  VectorParamsAs1DForOutWhenUnconnected=off
  wires:
  Divide/1 -> Multiply/1
  Sum/1 -> Divide/1
  In1/1 -> Sum/1
  Constant8/1 -> Sum2/1
  pwm_aileron_min/1 -> Sum1/2, Sum/2
  pwm_aileron_max/1 -> Sum1/1
  Multiply/1 -> Sum3/1
  Sum2/1 -> Multiply/2
  Constant9/1 -> Sum3/2, Sum2/2
  Sum1/1 -> Divide/2
  Sum3/1 -> Gain/1
  Gain/1 -> Saturation/1
  Saturation/1 -> Out1/1

== system PROVA_FINALE_LOAD_ARDUINO_15_10_RIF_COSTANTI/RADIOCOMANDO/ELEVATOR ==
  pwm_elevator_max : Inport
  In1 : Inport  Port=2
  pwm_elevator_min : Inport  Port=3
  Constant8 : Constant  Value=attuatore_Emax  OutDataTypeStr=double  SampleTime=-1
  Constant9 : Constant  Value=attuatore_Emin  OutDataTypeStr=double  SampleTime=-1
  Divide : Product  Inputs=*/
  Multiply : Product
  Sum : Sum  Inputs=|+-
  Sum1 : Sum  Inputs=|+-
  Sum2 : Sum  Inputs=|+-
  Sum3 : Sum  Inputs=|++
  Out1 : Outport  VectorParamsAs1DForOutWhenUnconnected=off
  wires:
  Sum3/1 -> Out1/1
  Multiply/1 -> Sum3/1
  Constant9/1 -> Sum3/2, Sum2/2
  Sum1/1 -> Divide/2
  Sum2/1 -> Multiply/2
  pwm_elevator_min/1 -> Sum1/2, Sum/2
  Constant8/1 -> Sum2/1
  pwm_elevator_max/1 -> Sum1/1
  Divide/1 -> Multiply/1
  In1/1 -> Sum/1
  Sum/1 -> Divide/1

== system PROVA_FINALE_LOAD_ARDUINO_15_10_RIF_COSTANTI/RADIOCOMANDO/ELEVATOR1 ==
  pwm_elevator_max : Inport
  In1 : Inport  Port=2
  pwm_elevator_min : Inport  Port=3
  Constant8 : Constant  Value=theta_max  OutDataTypeStr=double  SampleTime=-1
  Constant9 : Constant  Value=theta_min  OutDataTypeStr=double  SampleTime=-1
  Divide : Product  Inputs=*/
  Gain : Gain
  Multiply : Product
  Saturation : Saturate  UpperLimit=theta_max  LowerLimit=theta_min
  Sum : Sum  Inputs=|+-
  Sum1 : Sum  Inputs=|+-
  Sum2 : Sum  Inputs=|+-
  Sum3 : Sum  Inputs=|++
  Out1 : Outport  VectorParamsAs1DForOutWhenUnconnected=off
  wires:
  Sum3/1 -> Gain/1
  Multiply/1 -> Sum3/1
  Constant9/1 -> Sum3/2, Sum2/2
  Sum1/1 -> Divide/2
  Sum2/1 -> Multiply/2
  pwm_elevator_min/1 -> Sum1/2, Sum/2
  Constant8/1 -> Sum2/1
  pwm_elevator_max/1 -> Sum1/1
  Divide/1 -> Multiply/1
  In1/1 -> Sum/1
  Sum/1 -> Divide/1
  Gain/1 -> Saturation/1
  Saturation/1 -> Out1/1

== system PROVA_FINALE_LOAD_ARDUINO_15_10_RIF_COSTANTI/RADIOCOMANDO/RUDDER ==
  pwm_rudder_max : Inport
  In1 : Inport  Port=2
  pwm_rudder_min : Inport  Port=3
  Constant8 : Constant  Value=attuatore_Rmax  OutDataTypeStr=double  SampleTime=-1
  Constant9 : Constant  Value=attuatore_Rmin  OutDataTypeStr=double  SampleTime=-1
  Divide : Product  Inputs=*/
  Multiply : Product
  Sum1 : Sum  Inputs=|+-
  Sum2 : Sum  Inputs=|+-
  Sum3 : Sum  Inputs=|+-
  Sum4 : Sum  Inputs=|++
  Out1 : Outport  VectorParamsAs1DForOutWhenUnconnected=off
  wires:
  Divide/1 -> Multiply/1
  Sum2/1 -> Divide/2
  pwm_rudder_min/1 -> Sum1/2, Sum2/2
  Sum3/1 -> Multiply/2
  Multiply/1 -> Sum4/1
  Constant9/1 -> Sum4/2, Sum3/2
  Sum1/1 -> Divide/1
  Constant8/1 -> Sum3/1
  pwm_rudder_max/1 -> Sum2/1
  Sum4/1 -> Out1/1
  In1/1 -> Sum1/1

== system PROVA_FINALE_LOAD_ARDUINO_15_10_RIF_COSTANTI/RADIOCOMANDO/THROTTLE ==
  pwm_throttle_max : Inport
  In1 : Inport  Port=2
  pwm_throttle_min : Inport  Port=3
  Divide2 : Product  Inputs=*/
  Multiply1 : Product
  Sum2 : Sum  Inputs=|+-
  Sum3 : Sum  Inputs=|+-
  Sum4 : Sum  Inputs=|+-
  Sum5 : Sum  Inputs=|++
  manetta_massima : Constant  Value=attuatore_Tmax  OutDataTypeStr=double  SampleTime=-1
  manetta_minima : Constant  Value=attuatore_Tmin  OutDataTypeStr=double  SampleTime=-1
  Out1 : Outport  VectorParamsAs1DForOutWhenUnconnected=off
  wires:
  Sum4/1 -> Multiply1/2
  Divide2/1 -> Multiply1/1
  pwm_throttle_max/1 -> Sum3/1
  Sum3/1 -> Divide2/2
  Sum2/1 -> Divide2/1
  manetta_minima/1 -> Sum4/2, Sum5/2
  pwm_throttle_min/1 -> Sum3/2, Sum2/2
  In1/1 -> Sum2/1
  Multiply1/1 -> Sum5/1
  Sum5/1 -> Out1/1
  manetta_massima/1 -> Sum4/1

== system PROVA_FINALE_LOAD_ARDUINO_15_10_RIF_COSTANTI/Servi/AILERON1 ==
  pwm_aileron_max : Inport
  In1 : Inport  Port=2
  pwm-aileron_min : Inport  Port=3
  Constant : Constant  Value=attuatore_Amax  SampleTime=t_AP
  Constant1 : Constant  Value=attuatore_Amin  SampleTime=t_AP
  Divide : Product  Inputs=*/
  Multiply : Product
  Sum : Sum  Inputs=|+-
  Sum1 : Sum  Inputs=|+-
  Sum2 : Sum  Inputs=|+-
  Sum3 : Sum  Inputs=|++
  Out1 : Outport  VectorParamsAs1DForOutWhenUnconnected=off
  wires:
  Sum/1 -> Divide/1
  Constant1/1 -> Sum1/2, Sum/2
  In1/1 -> Sum/1
  Divide/1 -> Multiply/1
  Sum2/1 -> Multiply/2
  pwm-aileron_min/1 -> Sum2/2, Sum3/2
  Multiply/1 -> Sum3/1
  Sum3/1 -> Out1/1
  pwm_aileron_max/1 -> Sum2/1
  Constant/1 -> Sum1/1
  Sum1/1 -> Divide/2
